simulink model "auv_6dof_sim"  (R2016a)
settings: Solver=VariableStepAuto  StartTime=0.0  StopTime=100  RelTol=1e-3
libraries: simulink x6
settings Model: Creator=drew  LastModifiedBy=andrew
settings DataIOCC: LimitDataPoints=on
settings DebuggingCC: AllowSymbolicDim=off
settings ModelReferenceCC: PropagateSignalLabelsOutOfModel=off
settings GRTTargetCC: GeneratePreprocessorConditionals=Use local settings

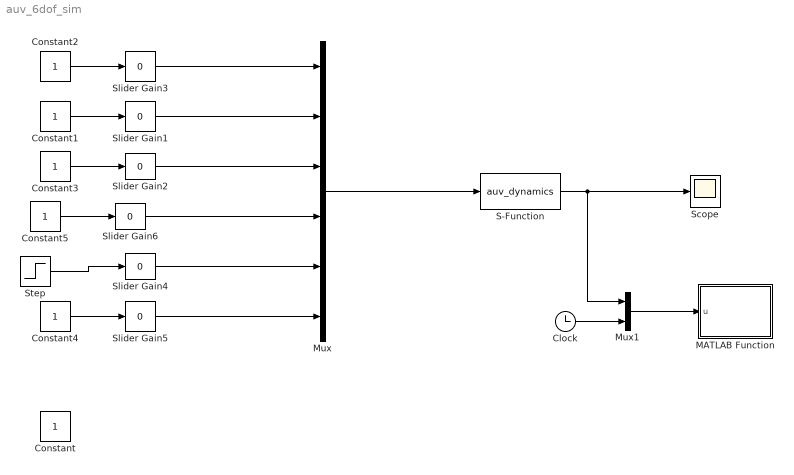
== system auv_6dof_sim ==
  Clock : Clock
  Constant{,1..5} (6 alike) : Constant
  MATLAB Function : MATLAB Function  TreatAsAtomicUnit=on
  Mux : Mux  Inputs=6
  Mux1 : Mux  Inputs=2
  S-Function : S-Function  FunctionName=auv_dynamics  Parameters=P  SFunctionDeploymentMode=off  EnableBusSupport=off
  Scope : Scope
  Slider Gain{1..6} (6 alike) : simulink/Math Operations/Slider Gain  low=-50  gain=0  high=50
  Step : Step  Time=3  Before=2  After=0  SampleTime=0
  wires:
  Constant3/1 -> Slider Gain2/1
  Constant1/1 -> Slider Gain1/1
  Constant4/1 -> Slider Gain5/1
  Step/1 -> Slider Gain4/1
  Slider Gain3/1 -> Mux/1
  Slider Gain1/1 -> Mux/2
  Slider Gain2/1 -> Mux/3
  Slider Gain6/1 -> Mux/4
  Slider Gain4/1 -> Mux/5
  Slider Gain5/1 -> Mux/6
  Mux/1 -> S-Function/1
  S-Function/1 -> Mux1/1, Scope/1
  Clock/1 -> Mux1/2
  Mux1/1 -> MATLAB Function/1(u)
  Constant2/1 -> Slider Gain3/1
  Constant5/1 -> Slider Gain6/1

== matlab function auv_6dof_sim/MATLAB Function ==
  data: u input
function drawAircraft(u) 
coder.extrinsic('patch')
pn = u(1);
pe = u(2);
pd = u(3);
ux = u(4);
vx = u(5);
wx = u(6);
phi = u(7);
theta = u(8);
psi = u(9);
p = u(10);
q = u(11);
r = u(12);

t = u(13);

persistent aircraftHandle

field_width = 10;
axis([ -10 10 -10 10 -10 10 ])
if isempty(aircraftHandle)
    figure(1), clf
    [V, F, patchcolors] = spacecraftVFC;
    
    XYZ = rotate(V', phi, theta, psi);
    
    %XYZ = translate(V, pn, pe, pd);
    
    R = [...
        0, 1, 0;...
        1, 0, 0;...
        0, 0, -1;...
        ];
    
    V = R*XYZ;
    
    aircraftHandle = patch('Vertices', V', 'Faces', F, ...
        'FaceVertexCData', patchcolors,...
        'FaceColor', 'flat',...
        'EraseMode', 'normal');
end

if t==0
            aircraftHandle = drawSpacecraftBody(pn, pe, pd, ...
                phi, theta, psi, aircraftHandle,'normal');
    
else
    aircraftHandle = drawSpacecraftBody(pn, pe, pd, ...
        phi, theta, psi, aircraftHandle,'normal');
end

function XYZ = rotate(XYZ,  phi, theta, psi)
R_roll = [...
    1, 0, 0; ...
    0, cos(phi), -sin(phi);...
    0, sin(phi), cos(phi)];
R_pitch = [...
    cos(theta), 0, sin(theta); ...
    0, 1, 0;...
    -sin(theta), 0, cos(theta)];

R_yaw = [...
    cos(psi), -sin(psi), 0; ...
    sin(psi), cos(psi), 0;...
    0, 0, 1];

R = R_roll * R_pitch * R_yaw;

XYZ = R * XYZ;
